simulink model "IEEE9_16b_2"  (R2020a)
settings: Solver=ode15s  StartTime=0.0  StopTime=5  MaxStep=1e-4  RelTol=1e-3
libraries: powerlib x35, sps_avr x3, simulink_extras x2, powerlib_meascontrol x2, simulink x1
settings Model: Creator=Pankaj  LastModifiedBy=ahmed
settings DataIOCC: ReturnWorkspaceOutputs=off
settings DebuggingCC: UnconnectedInputMsg=none  UnconnectedOutputMsg=none  UnconnectedLineMsg=none  ArithmeticOperatorsInVariantConditions=warning
settings SFSimCC: SimUseLocalCustomCode=off  CustomCodeUndefinedFunction=UseInterfaceOnly
settings RTWCC: RTWUseLocalCustomCode=off
settings CodeAppCC: StateflowObjectComments=on
settings SimscapeCC: SimscapeNormalizeSystem=off

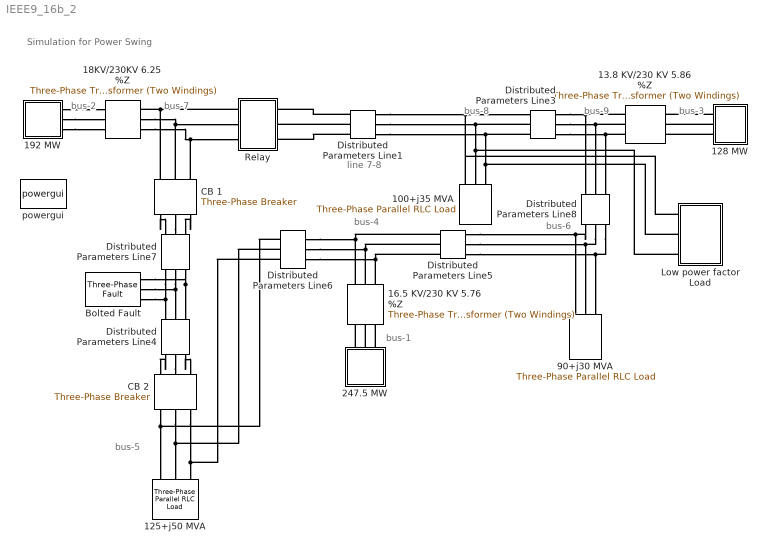
== system IEEE9_16b_2 ==
  note: Simulation for Power Swing
  note: bus-2
  note: bus-7
  note: bus-8
  note: bus-9
  note: bus-1
  note: bus-3
  note: bus-4
  note: bus-6
  note: bus-5
  note: line 7-8
  100+j35 MVA : powerlib/Elements/Three-Phase Parallel RLC Load  LConnTagsString=A|B|C  Configuration=Y (grounded)  NominalVoltage=(230000)*0.993698  Vabc=[1e3 1e3 1e3]  Vabcp=[1e3 1e3 1e3]  NominalFrequency=60  UnbalancedPower=off  ActivePower=100e6  InductivePower=35e6  CapacitivePower=0  Pabc=[10e3 9e3 11e3]  QLabc=[100 90 110]  QCabc=[100 90 110]  Pabcp=[10e3 9e3 11e3]  QLabcp=[100 90 110]  QCabcp=[100 90 110]  Measurements=None  LoadType=constant PQ
  125+j50 MVA : powerlib/Elements/Three-Phase Parallel RLC Load  LConnTagsString=A|B|C  Configuration=Y (grounded)  NominalVoltage=(223027)*1  Vabc=[1e3 1e3 1e3]  Vabcp=[1e3 1e3 1e3]  NominalFrequency=60  UnbalancedPower=off  ActivePower=125e6  InductivePower=50e6  CapacitivePower=0  Pabc=[10e3 9e3 11e3]  QLabc=[100 90 110]  QCabc=[100 90 110]  Pabcp=[10e3 9e3 11e3]  QLabcp=[100 90 110]  QCabcp=[100 90 110]  Measurements=None  LoadType=constant PQ
  128 MW : Subsystem
  13.8 KV/230 KV 5.86 %Z : powerlib/Elements/Three-Phase Transformer (Two Windings)  Winding1Connection=Yg  Winding2Connection=Yg  CoreType=Three single-phase transformers  SetSaturation=off  Hysteresis=off  DataFile='hysteresis'  SetInitialFlux=off  Measurements=None  UNITS=pu  NominalPower=[ 100e6 , 60 ]  Winding1=[13.8e3 , 1e-6 , 0 ]  Winding2=[ 230e3 , 1e-6, 0.0586 ]  Rm=500  Lm=500  L0=0.5  Saturation=[ 0,0 ; 0.0024,1.2 ; 1.0,1.52 ]  InitialFluxes=[ 0.8 , -0.8 , 0.7 ]  BreakLoop=off  DiscreteSolver=Trapezoidal iterative  DataType=off  TransfoNumber=1
  "16.5 KV/230 KV 5.76 %Z     " : powerlib/Elements/Three-Phase Transformer (Two Windings)  Winding1Connection=Yg  Winding2Connection=Yg  CoreType=Three single-phase transformers  SetSaturation=off  Hysteresis=off  DataFile='hysteresis'  SetInitialFlux=off  Measurements=None  UNITS=pu  NominalPower=[ 100e6 , 60 ]  Winding1=[16.5e3 , 1e-6, 0 ]  Winding2=[ 230e3 ,1e-6, 0.0576 ]  Rm=500  Lm=500  L0=0.5  Saturation=[ 0,0 ; 0.0024,1.2 ; 1.0,1.52 ]  InitialFluxes=[ 0.8 , -0.8 , 0.7 ]  BreakLoop=off  DiscreteSolver=Trapezoidal iterative  DataType=off  TransfoNumber=1
  18KV/230KV 6.25 %Z : powerlib/Elements/Three-Phase Transformer (Two Windings)  Winding1Connection=Yg  Winding2Connection=Yg  CoreType=Three single-phase transformers  SetSaturation=off  Hysteresis=off  DataFile='hysteresis'  SetInitialFlux=off  Measurements=None  UNITS=pu  NominalPower=[ 100e6 , 60 ]  Winding1=[ 18e3 , 1e-6 , 0]  Winding2=[ 230e3 , 1e-6, 0.0625 ]  Rm=500  Lm=500  L0=0.5  Saturation=[ 0,0 ; 0.0024,1.2 ; 1.0,1.52 ]  InitialFluxes=[ 0.8 , -0.8 , 0.7 ]  BreakLoop=off  DiscreteSolver=Trapezoidal iterative  DataType=off  TransfoNumber=1
  192 MW : Subsystem
  247.5 MW : Subsystem
  90+j30 MVA : powerlib/Elements/Three-Phase Parallel RLC Load  LConnTagsString=A|B|C  Configuration=Y (grounded)  NominalVoltage=(226177)*0.999999  Vabc=[1e3 1e3 1e3]  Vabcp=[1e3 1e3 1e3]  NominalFrequency=60  UnbalancedPower=off  ActivePower=90e6  InductivePower=30e6  CapacitivePower=0  Pabc=[10e3 9e3 11e3]  QLabc=[100 90 110]  QCabc=[100 90 110]  Pabcp=[10e3 9e3 11e3]  QLabcp=[100 90 110]  QCabcp=[100 90 110]  Measurements=None  LoadType=constant PQ
  Bolted Fault : powerlib/Elements/Three-Phase Fault  InitialStates=0  FaultA=on  FaultB=on  FaultC=on  GroundFault=off  SwitchTimes=0.2  External=off  SwitchStatus=NaN  FaultResistance=1e-6  GroundResistance=0.01  SnubberResistance=1e6  SnubberCapacitance=inf  Measurements=None
  CB 1 : powerlib/Elements/Three-Phase Breaker  InitialState=closed  SwitchA=on  SwitchB=on  SwitchC=on  SwitchTimes=3  External=off  BreakerResistance=0.01  SnubberResistance=1e6  SnubberCapacitance=inf  Measurements=None
  CB 2 : powerlib/Elements/Three-Phase Breaker  InitialState=closed  SwitchA=on  SwitchB=on  SwitchC=on  SwitchTimes=3  External=off  BreakerResistance=0.01  SnubberResistance=1e6  SnubberCapacitance=inf  Measurements=None
  Distributed Parameters Line1 : powerlib/Elements/Distributed Parameters Line  Phases=3  Frequency=60  Resistance=[0.044965 0.11241]  Inductance="[1.01e-3  2.02e-3]"  Capacitance=[12.74e-9 7.751e-9]  Length=100  x1=[-0.0004 -6.82796491334943e-09 72528.4160001859 -218588.479822374;-0.00035 -6.27008684641219e-09 76635.5741816138 -217182.598108978;-0.0003 -5.70998104747418e-09 80715.5041084443 -215699.552452614;-0.00025 -5.14784651945875e-09 84766.7562010016 -214139.869772342;-0.0002 -4.58388298608703e-09 88787.8910687075 -212504.104215993;-0.00015 -4.01829082091706e-09 92777.4800214907 -210792.836963279;-0.0001 -3.45127097615198e-09 96734.1055773932 -209006.676019307;-5e-05 -2.8830249112427e-09 100656.361966195 -207146.255998555]  x2=[-0.0004 -1.1431204063284e-08 62229.765747204 -219715.300074861;-0.00035 -1.09478361575261e-08 66359.9919840522 -218503.333092898;-0.0003 -1.04605785377109e-08 70466.6408317295 -217213.732917117;-0.00025 -9.96960432415053e-09 74548.2532174544 -215846.95773632;-0.0002 -9.47508795764522e-09 78603.3789637815 -214403.493159219;-0.00015 -8.97720513750531e-09 82630.577303842 -212883.852041907;-0.0001 -8.47613275912606e-09 86628.4173932417 -211288.574305635;-5e-05 -7.97204885113761e-09 90595.478818433 -209618.226744989]  x3=[-0.0004 2.47214142457228e-11 142.095952291051 -522.350151915625;-0.00035 2.45249559346704e-11 151.916197843285 -519.579075508434;-0.0003 2.43197840235529e-11 161.682468293792 -516.623395129752;-0.00025 2.41059714089733e-11 171.391293733184 -513.484160918744;-0.0002 2.38835940575356e-11 181.039224662013 -510.162488230377;-0.00015 2.36527309788538e-11 190.622833216359 -506.65955723914;-0.0001 2.34134641974804e-11 200.138714385737 -502.976612519736;-5e-05 2.31658787237637e-11 209.583487222877 -499.114962604885]  x4=[-0.0004 -6.81755980373169e-11 226.230187701687 -1047.93268485817;-0.00035 -6.60199840333111e-11 245.941825546425 -1043.48242296301;-0.0003 -6.38409134433403e-11 265.566081431627 -1038.66141673164;-0.00025 -6.16391604808091e-11 285.095982952621 -1033.47137904461;-0.0002 -5.94155074180612e-11 304.52459122839 -1027.91415389759;-0.00015 -5.71707443084416e-11 323.845003366925 -1021.99171574624;-0.0001 -5.49056687055944e-11 343.05035491779 -1015.70616880461;-5e-05 -5.2621085380096e-11 362.133822311028 -1009.05974629762]  x5=0.000395689524753941  V1=ones(3,3)  V2=ones(3,3)  I1=ones(3,3)  I2=ones(3,3)  nHarmo=1  Measurements=None
  Distributed Parameters Line3 : powerlib/Elements/Distributed Parameters Line  Phases=3  Frequency=60  Resistance=[ 0.062951 0.15737]  Inductance="[ 1.414e-3  3.53e-3]"  Capacitance=[12.74e-9 7.751e-9]  Length=100  x1=[-0.00055 -1.2856259388639e-08 0 0;-0.0005 -1.23855852223811e-08 0 0;-0.00045 -1.19105105166692e-08 58077.4295709002 -220849.203256907;-0.0004 -1.1431204063284e-08 62229.765747204 -219715.300074861;-0.00035 -1.09478361575261e-08 66359.9919840522 -218503.333092898;-0.0003 -1.04605785377109e-08 70466.6408317295 -217213.732917117;-0.00025 -9.96960432415053e-09 74548.2532174544 -215846.95773632;-0.0002 -9.47508795764522e-09 78603.3789637815 -214403.493159219;-0.00015 -8.97720513750531e-09 82630.577303842 -212883.852041907;-0.0001 -8.47613275912606e-09 86628.4173932417 -211288.574305635;-5e-05 -7.97204885113761e-09 90595.478818433 -209618.226744989]  x2=[-0.00055 -1.49760945438105e-08 0 0;-0.0005 -1.45496058699479e-08 0 0;-0.00045 -1.41179477903994e-08 67158.9011993995 -221165.376830188;-0.0004 -1.36812736712252e-08 71315.5829852004 -219860.246936089;-0.00035 -1.32397386606606e-08 75446.9266839443 -218477.001743144;-0.0003 -1.27934996339924e-08 79551.4644488867 -217016.132711783;-0.00025 -1.23427151378221e-08 83627.7379573042 -215478.158881818;-0.0002 -1.18875453337346e-08 87674.2989286288 -213863.626688027;-0.00015 -1.14281519413939e-08 91689.7096390155 -212173.109766011;-0.0001 -1.0964698181085e-08 95672.543432159 -210407.208748382;-5e-05 -1.04973487157221e-08 99621.385226177 -208566.551051363]  x3=[-0.00055 -6.89304608922042e-12 0 0;-0.0005 -6.57772896748363e-12 0 0;-0.00045 -6.26007480996533e-12 133.037448642828 -835.2647228767;-0.0004 -5.94019647767513e-12 148.757241469557 -832.60880210302;-0.00035 -5.61820762186136e-12 164.424181556718 -829.657059386518;-0.0003 -5.2942226436313e-12 180.032702515096 -826.410543467325;-0.00025 -4.96835665330503e-12 195.577258711518 -822.870407817091;-0.0002 -4.64072542951725e-12 211.052327239184 -819.037910229153;-0.00015 -4.31144537808173e-12 226.452409879932 -814.914412371656;-0.0001 -3.98063349063283e-12 241.77203505773 -810.501379303756;-5e-05 -3.64840730305896e-12 257.005759782698 -805.800378955086]  x4=[-0.00055 -4.04271531251667e-11 0 0;-0.0005 -3.95164976157587e-11 0 0;-0.00045 -3.85918020829103e-11 132.207750255798 -502.668253747127;-0.0004 -3.76533950665412e-11 141.658729090772 -500.087037974906;-0.00035 -3.67016099781961e-11 151.059377253824 -497.328143659317;-0.0003 -3.57367849825848e-11 160.406354739424 -494.392551022371;-0.00025 -3.4759262877434e-11 169.69634061098 -491.281303066156;-0.0002 -3.37693909716933e-11 178.926034180746 -487.995505202256;-0.00015 -3.27675209621373e-11 188.092156182545 -484.536324859005;-0.0001 -3.17540088084098e-11 197.191449936875 -480.904991066709;-5e-05 -3.07292146065531e-11 206.220682507993 -477.102794020972]  x5=0.000523077718890797  V1=ones(3,3)  V2=ones(3,3)  I1=ones(3,3)  I2=ones(3,3)  nHarmo=1  Measurements=None
  Distributed Parameters Line4 : powerlib/Elements/Distributed Parameters Line  Phases=3  Frequency=60  Resistance=[ 0.16928 0.4232]  Inductance="[ 2.259e-3  5.64e-3]"  Capacitance=[12.74e-9 7.751e-9]  Length=80  x1=[-0.00055 -1.40561812794253e-08 0 0;-0.0005 -1.36829660387334e-08 0 0;-0.00045 -1.33048893053609e-08 48295.948807218 -217554.641827645;-0.0004 -1.29220854081711e-08 52387.9255838606 -216605.688790323;-0.00035 -1.25346903555658e-08 56461.2891799944 -215579.776783167;-0.0003 -1.21428417871626e-08 60514.5923489297 -214477.270307828;-0.00025 -1.1746678924892e-08 64546.3949713508 -213298.561079608;-0.0002 -1.13463425235325e-08 68555.2645669839 -212044.067888283;-0.00015 -1.09419748207014e-08 72539.7768035502 -210714.23644931;-0.0001 -1.0533719486318e-08 76498.516002825 -209309.539245467;-5e-05 -1.01217215715586e-08 80430.0756436207 -207830.475358982]  x2=[-0.00055 -6.92029081309933e-09 0 0;-0.0005 -6.32833411269307e-09 0 0;-0.00045 -5.73412898530969e-09 64426.420227431 -220200.980450415;-0.0004 -5.13788654920156e-09 68565.4107597344 -218947.522559977;-0.00035 -4.53981864646715e-09 72680.0403280773 -217616.273657318;-0.0003 -3.94013776778453e-09 76768.8470241662 -216207.706728834;-0.00025 -3.33905697691445e-09 80830.3781144513 -214722.322231648;-0.0002 -2.73678983499979e-09 84863.1905562757 -213160.647915798;-0.00015 -2.1335503246883e-09 88865.8515105816 -211523.238636734;-0.0001 -1.52955277410559e-09 92836.938850991 -209810.676158175;-5e-05 -9.25011780705398e-10 96775.0416690807 -208023.568945415]  x3=[-0.00055 -7.55288067688039e-11 0 0;-0.0005 -7.41259584887901e-11 0 0;-0.00045 -7.26967736086847e-11 78.3022662123242 -745.938765685069;-0.0004 -7.12417599110705e-11 92.3481089992822 -744.330373079888;-0.00035 -6.97614343553859e-11 106.361140942839 -742.457523437368;-0.0003 -6.82563228942521e-11 120.33638327947 -740.32088217207;-0.00025 -6.67269602866046e-11 134.268870672118 -737.921208422462;-0.0002 -6.51738899076954e-11 148.153652974353 -735.2593547812;-0.00015 -6.35976635560353e-11 161.985796989138 -732.336266992209;-0.0001 -6.19988412573415e-11 175.760388221566 -729.152983614661;-5e-05 -6.03779910655638e-11 189.472532624964 -725.710635653982]  x4=[-0.00055 4.56513386616241e-11 0 0;-0.0005 4.5308230221681e-11 0 0;-0.00045 4.49490239832806e-11 100.066822114028 -290.202191891929;-0.0004 4.45738475706891e-11 105.51888972623 -288.264531923678;-0.00035 4.41828342822994e-11 110.933466979353 -286.224452939841;-0.0003 4.37761230432709e-11 116.308630099881 -284.082679770765;-0.00025 4.33538583561703e-11 121.642469317951 -281.83997337826;-0.0002 4.29161902496303e-11 126.933089545888 -279.497130585228;-0.00015 4.24632742250451e-11 132.178611051516 -277.054983792557;-0.0001 4.19952712013217e-11 137.377170126022 -274.514400683375;-5e-05 4.15123474577058e-11 142.526919746119 -271.876283914763]  x5=0.000528942431650175  V1=ones(3,3)  V2=ones(3,3)  I1=ones(3,3)  I2=ones(3,3)  nHarmo=1  Measurements=None
  Distributed Parameters Line5 : powerlib/Elements/Distributed Parameters Line  Phases=3  Frequency=60  Resistance=[ 0.08993 0.224825]  Inductance="[ 1.29e-3  3.22e-3]"  Capacitance=[12.74e-9 7.751e-9]  Length=100  x1=[-0.0005 -1.54417229393186e-08 59227.4468730644 -220964.294919318;-0.00045 -1.50769173300264e-08 63381.7481353212 -219808.693934478;-0.0004 -1.47067549637975e-08 67513.5301642651 -218574.995967328;-0.00035 -1.43313673575578e-08 71621.3249574154 -217263.639344882;-0.0003 -1.39508878847366e-08 75703.6730348416 -215875.089985903;-0.00025 -1.35654517278786e-08 79759.1239577106 -214409.841235366;-0.0002 -1.31751958306153e-08 83786.2368436198 -212868.413689177;-0.00015 -1.27802588490086e-08 87783.5808785366 -211251.355009202;-0.0001 -1.23807811022875e-08 91749.7358251591 -209559.23972869;-5e-05 -1.19769045229934e-08 95683.2925275201 -207792.669048144]  x2=[-0.0005 -1.64800198971184e-08 47810.7569296928 -220880.136660959;-0.00045 -1.61471045841858e-08 51965.4999610341 -219939.738829347;-0.0004 -1.58084522818807e-08 56101.7798976792 -218921.197455797;-0.00035 -1.54641833117536e-08 60218.1271390618 -217824.874423211;-0.0003 -1.51144199909305e-08 64313.0791666077 -216651.159249941;-0.00025 -1.47592865886536e-08 68385.18106336 -215400.4689514;-0.0002 -1.43989092821299e-08 72432.9860309045 -214073.247891895;-0.00015 -1.40334161117004e-08 76455.0559034106 -212669.967626748;-0.0001 -1.36629369353481e-08 80449.9616586038 -211191.126734758;-5e-05 -1.32876033825604e-08 84416.2839254919 -209637.25064105]  x3=[-0.0005 -1.39450438340109e-11 90.110530585494 -468.848251260046;-0.00045 -1.36379171260647e-11 98.9315787794445 -467.06652149822;-0.0004 -1.33259449311022e-11 107.717477054529 -465.118845225298;-0.00035 -1.30092380913587e-11 116.465103822925 -463.005914441386;-0.0003 -1.26879091312664e-11 125.171351094496 -460.72847986073;-0.00025 -1.23620722174747e-11 133.833125581041 -458.287350644992;-0.0002 -1.20318431182876e-11 142.447349795329 -455.68339411576;-0.00015 -1.16973391625316e-11 151.010963144515 -452.917535446389;-0.0001 -1.13586791978694e-11 159.520923017552 -449.990757333293;-5e-05 -1.1015983548574e-11 167.974205866218 -446.904099646802]  x4=[-0.0005 -3.93672360983282e-11 134.386791841113 -915.942580841835;-0.00045 -3.87069965166257e-11 151.626950313248 -913.246876554873;-0.0004 -3.80330045233687e-11 168.813236451926 -910.226700001204;-0.00035 -3.73454995847032e-11 185.939544051518 -906.883124235176;-0.0003 -3.66447259678603e-11 202.999788216481 -903.217337213338;-0.00025 -3.59309326543691e-11 219.987907523298 -899.230641372365;-0.0002 -3.52043732515953e-11 236.89786617407 -894.924453166305;-0.00015 -3.44653059026349e-11 253.723656141008 -890.300302563323;-0.0001 -3.3713993194598e-11 270.459299301054 -885.35983250211;-5e-05 -3.29507020653121e-11 287.098849559883 -880.104798308154]  x5=0.000499582025297148  V1=ones(3,3)  V2=ones(3,3)  I1=ones(3,3)  I2=ones(3,3)  nHarmo=1  Measurements=None
  Distributed Parameters Line6 : powerlib/Elements/Distributed Parameters Line  Phases=3  Frequency=60  Resistance=[ 0.0529 0.13225]  Inductance="[ 1.192e-3  2.38e-3]"  Capacitance=[12.74e-9 7.751e-9]  Length=100  x1=[-0.00045 -1.33671750716869e-08 0 0;-0.0004 -1.29840046537664e-08 52388.2213168269 -216603.227745078;-0.00035 -1.25962210808172e-08 56461.5384736403 -215577.310601006;-0.0003 -1.22039621304964e-08 60514.7951146823 -214474.799864975;-0.00025 -1.18073671705413e-08 64546.5511371684 -213296.087253798;-0.0002 -1.14065771092526e-08 68555.3740773815 -212041.591558455;-0.00015 -1.10017343454308e-08 72539.8396196194 -210711.758495291;-0.0001 -1.05929827177822e-08 76498.5321022475 -209307.060547664;-5e-05 -1.01804674538136e-08 80430.0450206764 -207827.996798064]  x2=[-0.00045 -1.50769173300264e-08 0 0;-0.0004 -1.47067549637975e-08 67513.5301642651 -218574.995967328;-0.00035 -1.43313673575578e-08 71621.3249574154 -217263.639344882;-0.0003 -1.39508878847366e-08 75703.6730348416 -215875.089985903;-0.00025 -1.35654517278786e-08 79759.1239577106 -214409.841235366;-0.0002 -1.31751958306153e-08 83786.2368436198 -212868.413689177;-0.00015 -1.27802588490086e-08 87783.5808785366 -211251.355009202;-0.0001 -1.23807811022875e-08 91749.7358251591 -209559.23972869;-5e-05 -1.19769045229934e-08 95683.2925275201 -207792.669048144]  x3=[-0.00045 -2.14191175718911e-11 0 0;-0.0004 -2.11528317147279e-11 113.045801628693 -1046.87113054036;-0.00035 -2.08790303571782e-11 132.757560724253 -1044.55441681095;-0.0003 -2.05978107795606e-11 152.422151690629 -1041.86657787103;-0.00025 -2.03092728978519e-11 172.032587792285 -1038.80856869695;-0.0002 -2.00135192281876e-11 191.581901534652 -1035.38147578482;-0.00015 -1.97106548504382e-11 211.063147139644 -1031.58651676444;-0.0001 -1.94007873708751e-11 230.469403013459 -1027.42503996668;-5e-05 -1.90840268839383e-11 249.79377420579 -1022.89852394442]  x4=[-0.00045 -3.48518737560347e-11 0 0;-0.0004 -3.3860723191614e-11 170.092694709932 -386.073129797578;-0.00035 -3.28575420734751e-11 177.339340108603 -382.798555495363;-0.0003 -3.18426868270926e-11 184.522977684155 -379.387974689121;-0.00025 -3.08165180257032e-11 191.641055124364 -375.842599141972;-0.0002 -2.97794002621957e-11 198.691043410209 -372.163688508968;-0.00015 -2.87317020195732e-11 205.670437714421 -368.352549889537;-0.0001 -2.76737955400325e-11 212.576758291438 -364.410537363085;-5e-05 -2.66060566927085e-11 219.407551358443 -360.339051507892]  x5=0.000429504132692574  V1=ones(3,3)  V2=ones(3,3)  I1=ones(3,3)  I2=ones(3,3)  nHarmo=1  Measurements=None
  Distributed Parameters Line7 : powerlib/Elements/Distributed Parameters Line  Phases=3  Frequency=60  Resistance=[ 0.16928 0.4232]  Inductance="[ 2.259e-3  5.64e-3]"  Capacitance=[12.74e-9 7.751e-9]  Length=20  x1=[-0.00015 -2.13190541884307e-09 88865.8515105816 -211523.238636734;-0.0001 -1.52845584541928e-09 92836.938850991 -209810.676158175;-5e-05 -9.24463218911547e-10 96775.0416690807 -208023.568945415]  x2=[-0.00015 -4.00540707204123e-09 92776.5259316086 -210790.754370917;-0.0001 -3.43782632914382e-09 96733.1124034512 -209004.611780059;-5e-05 -2.86902414292128e-09 100655.330061063 -207144.210845835]  x3=[-0.00015 2.91772913405599e-11 284.591423982608 -715.419057494935;-0.0001 2.89453628397094e-11 298.025372274848 -709.927849901303;-5e-05 2.87031501892687e-11 311.353433571401 -704.184408323007]  x4=[-0.00015 -3.97589260516673e-11 123.975117525793 -290.153181832622;-0.0001 -3.81522539820278e-11 129.422014019475 -287.764895368002;-5e-05 -3.65320265982149e-11 134.822927487834 -285.274367406284]  x5=0.000132235607912544  V1=ones(3,3)  V2=ones(3,3)  I1=ones(3,3)  I2=ones(3,3)  nHarmo=1  Measurements=None
  Distributed Parameters Line8 : powerlib/Elements/Distributed Parameters Line  Phases=3  Frequency=60  Resistance=[ 0.20631 0.5157]  Inductance="[ 2.38e-3  6.09e-3]"  Capacitance=[12.74e-9 7.751e-9]  Length=100  x1=[-0.0007 -1.77519770428368e-08 31036.7644346723 -223854.029074571;-0.00065 -1.74431715104659e-08 35250.5405219156 -223229.267237956;-0.0006 -1.71281685023151e-08 39451.792259961 -222525.193105624;-0.00055 -1.68070799374532e-08 43639.0269640709 -221742.056831762;-0.0005 -1.64800198971184e-08 47810.7569296928 -220880.136660959;-0.00045 -1.61471045841858e-08 51965.4999610341 -219939.738829347;-0.0004 -1.58084522818807e-08 56101.7798976792 -218921.197455797;-0.00035 -1.54641833117536e-08 60218.1271390618 -217824.874423211;-0.0003 -1.51144199909305e-08 64313.0791666077 -216651.159249941;-0.00025 -1.47592865886536e-08 68385.18106336 -215400.4689514;-0.0002 -1.43989092821299e-08 72432.9860309045 -214073.247891895;-0.00015 -1.40334161117004e-08 76455.0559034106 -212669.967626748;-0.0001 -1.36629369353481e-08 80449.9616586038 -211191.126734758;-5e-05 -1.32876033825604e-08 84416.2839254919 -209637.25064105]  x2=[-0.0007 -1.62230383430129e-08 46047.3963086879 -226504.047430459;-0.00065 -1.58129594474007e-08 50308.4541681047 -225595.888989612;-0.0006 -1.53972622825922e-08 54551.6376733053 -224607.577403608;-0.00055 -1.49760945438105e-08 58775.4392413945 -223539.463814848;-0.0005 -1.45496058699479e-08 62978.3581757875 -222391.927719005;-0.00045 -1.41179477903994e-08 67158.9011993995 -221165.376830188;-0.0004 -1.36812736712252e-08 71315.5829852005 -219860.246936089;-0.00035 -1.32397386606606e-08 75446.9266839443 -218477.001743144;-0.0003 -1.27934996339924e-08 79551.4644488867 -217016.132711783;-0.00025 -1.23427151378221e-08 83627.7379573042 -215478.158881818;-0.0002 -1.18875453337346e-08 87674.2989286288 -213863.626688027;-0.00015 -1.14281519413939e-08 91689.7096390155 -212173.109766011;-0.0001 -1.0964698181085e-08 95672.543432159 -210407.208748382;-5e-05 -1.04973487157221e-08 99621.385226177 -208566.551051363]  x3=[-0.0007 -4.18504150647578e-11 24.6100303573918 -669.614087088405;-0.00065 -4.13572954088089e-11 37.2268292493843 -669.031279274382;-0.0006 -4.08494817027289e-11 49.8304016262044 -668.210767832504;-0.00055 -4.03271543703095e-11 62.4162694986001 -667.152844286579;-0.0005 -3.97904989919648e-11 74.9799611676454 -665.857884511807;-0.00045 -3.92397062387955e-11 87.5170128135137 -664.326348601228;-0.0004 -3.8674971804844e-11 100.022970081452 -662.55878070226;-0.00035 -3.80964963375657e-11 112.493389664392 -660.55580882336;-0.0003 -3.75044853665396e-11 124.923840881634 -658.318144610899;-0.00025 -3.68991492304449e-11 137.30990725305 -655.846583096318;-0.0002 -3.62807030023282e-11 149.647188068237 -653.142002413653;-0.00015 -3.56493664131896e-11 161.931299950067 -650.205363487544;-0.0001 -3.50053637739131e-11 174.157878412078 -647.037709691817;-5e-05 -3.43489238955698e-11 186.322579409164 -643.640166478783]  x4=[-0.0007 5.14626612385657e-14 41.4725891803423 -353.789217989042;-0.00065 2.35381322552756e-13 48.1335635245818 -352.944672963745;-0.0006 4.1921635400384e-13 54.7774362428946 -351.974728376731;-0.00055 6.02902439880495e-13 61.4018467989396 -350.879728844695;-0.0005 7.86374317391051e-13 68.0044415711891 -349.660063415755;-0.00045 9.69566799851051e-13 74.5828746891595 -348.316165431231;-0.0004 1.15241479984377e-12 81.134808866888 -346.848512371678;-0.00035 1.33485335234547e-12 87.6579162333591 -345.257625687239;-0.0003 1.51681763780714e-12 94.149879159586 -343.544070612379;-0.00025 1.6982430051846e-12 100.608391082053 -341.708455965056;-0.0002 1.8790649949087e-12 107.031157322228 -339.751433930413;-0.00015 2.05921936178751e-12 113.415895901847 -337.673699829062;-0.0001 2.23864209783228e-12 119.760338353696 -335.475991870034;-5e-05 2.41726945499926e-12 126.06223052758 -333.159090888504]  x5=0.000687048688231045  V1=ones(3,3)  V2=ones(3,3)  I1=ones(3,3)  I2=ones(3,3)  nHarmo=1  Measurements=None
  Low power factor Load : Subsystem
  Relay : Subsystem
  powergui : powerlib/powergui  Priority=1  SimulationMode=Discrete  SampleTime=50e-6  frequency=60  Iterations=50  frequencyindice=60  Pbase=100e6  ErrMax=0.0001  UnitsV=kV  UnitsW=MW  buscounter=0  FunctionMessages=off  echomessages=off  EnableUseOfTLC=off  CurrentSourceSwitches=off  DisableSnubberDevices=off  DisableRonSwitches=off  DisableVfSwitches=off  DisplayEquations=off  AutomaticDiscreteSolvers=off  SolverType=Tustin/Backward Euler (TBE)  Interpol=off  ExternalGateDelay=off  methode=off  Ts=100  x0status=blocks  SPID=on  SwTol=0  HookPort=off  NonlinearTolerance=1e-4  nMaxIteration=100  ContinueOnMaxIteration=off  RestoreLinks=warning  ResistiveCurrentMeasurement=off  Frange=[0:2:500]  Ylog=off  Xlog=on  ShowGrid=off  save=off  variable=ZData  structure=0  ZoomFFT=off  StartTime=0.0  cycles=1  DisplayStyle=1  fundamental=60  FreqAxis=off  MaxFrequency=1000  frequencyindicesteady=1  RmsSteady=1  display=off
  connections:
  Distributed Parameters Line1/RConn1 -- 100+j35 MVA/LConn1 -- Low power factor Load/RConn1 -- Distributed Parameters Line3/LConn1
  Distributed Parameters Line1/RConn2 -- Low power factor Load/RConn3 -- 100+j35 MVA/LConn2 -- Distributed Parameters Line3/LConn2
  Distributed Parameters Line1/RConn3 -- Distributed Parameters Line3/LConn3 -- 100+j35 MVA/LConn3 -- Low power factor Load/RConn2
  Distributed Parameters Line5/RConn1 -- Distributed Parameters Line8/LConn1 -- 90+j30 MVA/LConn1
  Distributed Parameters Line5/RConn3 -- Distributed Parameters Line8/LConn3 -- 90+j30 MVA/LConn3
  Distributed Parameters Line3/RConn1 -- 13.8 KV/230 KV 5.86 %Z/RConn1 -- Distributed Parameters Line8/RConn1
  Distributed Parameters Line3/RConn2 -- 13.8 KV/230 KV 5.86 %Z/RConn2 -- Distributed Parameters Line8/RConn2
  Distributed Parameters Line3/RConn3 -- 13.8 KV/230 KV 5.86 %Z/RConn3 -- Distributed Parameters Line8/RConn3
  Relay/LConn1 -- CB 1/RConn1 -- 18KV/230KV 6.25 %Z/RConn1
  18KV/230KV 6.25 %Z/RConn2 -- CB 1/RConn2 -- Relay/LConn2
  18KV/230KV 6.25 %Z/RConn3 -- Relay/LConn3 -- CB 1/RConn3
  Distributed Parameters Line5/RConn2 -- Distributed Parameters Line8/LConn2 -- 90+j30 MVA/LConn2
  Distributed Parameters Line6/RConn1 -- Distributed Parameters Line5/LConn1 -- "16.5 KV/230 KV 5.76 %Z     "/RConn1
  Distributed Parameters Line6/RConn2 -- Distributed Parameters Line5/LConn2 -- "16.5 KV/230 KV 5.76 %Z     "/RConn2
  Distributed Parameters Line6/RConn3 -- Distributed Parameters Line5/LConn3 -- "16.5 KV/230 KV 5.76 %Z     "/RConn3
  247.5 MW/RConn1 -- "16.5 KV/230 KV 5.76 %Z     "/LConn1
  247.5 MW/RConn2 -- "16.5 KV/230 KV 5.76 %Z     "/LConn2
  247.5 MW/RConn3 -- "16.5 KV/230 KV 5.76 %Z     "/LConn3
  128 MW/RConn1 -- 13.8 KV/230 KV 5.86 %Z/LConn1
  128 MW/RConn2 -- 13.8 KV/230 KV 5.86 %Z/LConn2
  128 MW/RConn3 -- 13.8 KV/230 KV 5.86 %Z/LConn3
  192 MW/RConn1 -- 18KV/230KV 6.25 %Z/LConn1
  192 MW/RConn2 -- 18KV/230KV 6.25 %Z/LConn2
  192 MW/RConn3 -- 18KV/230KV 6.25 %Z/LConn3
  Distributed Parameters Line1/LConn1 -- Relay/RConn1
  Distributed Parameters Line1/LConn2 -- Relay/RConn2
  Distributed Parameters Line1/LConn3 -- Relay/RConn3
  Distributed Parameters Line7/LConn1 -- Distributed Parameters Line4/RConn1 -- Bolted Fault/LConn1
  Distributed Parameters Line7/LConn2 -- Distributed Parameters Line4/RConn2 -- Bolted Fault/LConn2
  Distributed Parameters Line7/LConn3 -- Distributed Parameters Line4/RConn3 -- Bolted Fault/LConn3
  CB 1/LConn2 -- Distributed Parameters Line7/RConn2
  CB 1/LConn1 -- Distributed Parameters Line7/RConn1
  CB 1/LConn3 -- Distributed Parameters Line7/RConn3
  Distributed Parameters Line4/LConn2 -- CB 2/RConn2
  Distributed Parameters Line4/LConn1 -- CB 2/RConn1
  Distributed Parameters Line4/LConn3 -- CB 2/RConn3
  CB 2/LConn2 -- Distributed Parameters Line6/LConn2 -- 125+j50 MVA/LConn2
  CB 2/LConn1 -- Distributed Parameters Line6/LConn1 -- 125+j50 MVA/LConn1
  CB 2/LConn3 -- Distributed Parameters Line6/LConn3 -- 125+j50 MVA/LConn3

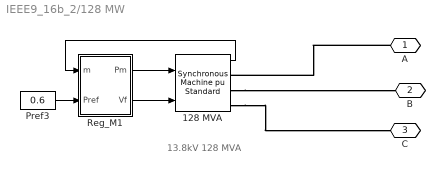
== system IEEE9_16b_2/128 MW ==
  note: 13.8kV 128 MVA
  128 MVA : powerlib/Machines/Synchronous Machine pu Standard  PresetModel=No  MechanicalLoad=Mechanical power Pm  ShowDetailedParameters=on  RotorType=Salient-pole  Units=per unit standard parameters  MeasurementBus=off  NominalParameters="[128e6  13800   60 ]"  Reactances1=[ 31 32 33 34 35 36 37 ]  Reactances2=[ 1.305, 0.296, 0.252, 0.474, 0.243, 0.18 ]  dAxisTimeConstants=Short-circuit  qAxisTimeConstants=Open-circuit  TimeConstants1=[]  TimeConstants2=[]  TimeConstants3=[]  TimeConstants4=[]  TimeConstants5=[ 1.01, 0.053, 0.1 ]  TimeConstants6=[]  TimeConstants7=[]  TimeConstants8=[]  StatorResistance=2.8544e-3  Mechanical="[20 0  32]"  PolePairs=32  InitialConditions=[0 -74.5248 0.603223 0.603223 0.603223 5.08525 -114.915 125.085 1.10339]  SetSaturation=off  Saturation=[0.6404,0.7127,0.8441,0.9214,0.9956,1.082,1.19,1.316,1.457;0.7,0.7698,0.8872,0.9466,0.9969,1.046,1.1,1.151,1.201]  LoadFlowParameters=[1 500000000 0 0 0]  TsPowergui=0  TsBlock=-1  IterativeModel=Trapezoidal non iterative  IterativeDiscreteModel=Trapezoidal non iterative  BusType=PV  Pref=0.6*128e6  Qref=0  Qmin=-Inf  Qmax=Inf  PLF=0  QLF=0
      settings: AttributesFormatString=\n\n
  Pref3 : Constant  Value=0.6
  Reg_M1 : Subsystem
  A : PMIOPort  Side=Right
  B : PMIOPort  Port=2  Side=Right
  C : PMIOPort  Port=3  Side=Right
  wires:
  Reg_M1/1(Pm) -> 128 MVA/1
  Reg_M1/2(Vf) -> 128 MVA/2
  Pref3/1 -> Reg_M1/2(Pref)
  128 MVA/1 -> Reg_M1/1(m)
  connections:
  A/RConn1 -- 128 MVA/RConn1
  128 MVA/RConn2 -- B/RConn1
  128 MVA/RConn3 -- C/RConn1

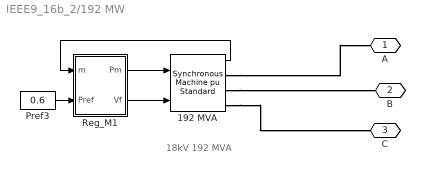
== system IEEE9_16b_2/192 MW ==
  note: 18kV 192 MVA
  192 MVA : powerlib/Machines/Synchronous Machine pu Standard  PresetModel=No  MechanicalLoad=Mechanical power Pm  ShowDetailedParameters=on  RotorType=Salient-pole  Units=per unit standard parameters  MeasurementBus=off  NominalParameters="[192e6  18000   60 ]"  Reactances1=[ 31 32 33 34 35 36 37 ]  Reactances2=[ 1.305, 0.296, 0.252, 0.474, 0.243, 0.18 ]  dAxisTimeConstants=Short-circuit  qAxisTimeConstants=Open-circuit  TimeConstants1=[]  TimeConstants2=[]  TimeConstants3=[]  TimeConstants4=[]  TimeConstants5=[ 1.01, 0.053, 0.1 ]  TimeConstants6=[]  TimeConstants7=[]  TimeConstants8=[]  StatorResistance=2.8544e-3  Mechanical="[20 0  32]"  PolePairs=32  InitialConditions=[0 -73.0594 0.600015 0.600015 0.600015 0.71576 -119.284 120.716 1.18255]  SetSaturation=off  Saturation=[0.6404,0.7127,0.8441,0.9214,0.9956,1.082,1.19,1.316,1.457;0.7,0.7698,0.8872,0.9466,0.9969,1.046,1.1,1.151,1.201]  LoadFlowParameters=[1 500000000 0 0 0]  TsPowergui=0  TsBlock=-1  IterativeModel=Trapezoidal non iterative  IterativeDiscreteModel=Trapezoidal non iterative  BusType=PV  Pref=0.6*192e6  Qref=0  Qmin=-Inf  Qmax=Inf  PLF=0  QLF=0
      settings: AttributesFormatString=\n\n
  Pref3 : Constant  Value=0.6
  Reg_M1 : Subsystem
  A : PMIOPort  Side=Right
  B : PMIOPort  Port=2  Side=Right
  C : PMIOPort  Port=3  Side=Right
  wires:
  Reg_M1/1(Pm) -> 192 MVA/1
  192 MVA/1 -> Reg_M1/1(m)
  Reg_M1/2(Vf) -> 192 MVA/2
  Pref3/1 -> Reg_M1/2(Pref)
  connections:
  192 MVA/RConn1 -- A/RConn1
  192 MVA/RConn3 -- C/RConn1
  192 MVA/RConn2 -- B/RConn1

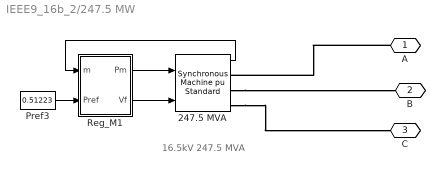
== system IEEE9_16b_2/247.5 MW ==
  note: 16.5kV 247.5 MVA
  247.5 MVA : powerlib/Machines/Synchronous Machine pu Standard  PresetModel=No  MechanicalLoad=Mechanical power Pm  ShowDetailedParameters=on  RotorType=Salient-pole  Units=per unit standard parameters  MeasurementBus=off  NominalParameters="[247.5e6  16500   60 ]"  Reactances1=[ 31 32 33 34 35 36 37 ]  Reactances2=[ 1.305, 0.296, 0.252, 0.474, 0.243, 0.18 ]  dAxisTimeConstants=Short-circuit  qAxisTimeConstants=Open-circuit  TimeConstants1=[]  TimeConstants2=[]  TimeConstants3=[]  TimeConstants4=[]  TimeConstants5=[ 1.01, 0.053, 0.1 ]  TimeConstants6=[]  TimeConstants7=[]  TimeConstants8=[]  StatorResistance=2.8544e-3  Mechanical=[20 0 32]  PolePairs=32  InitialConditions=[0 -76.6925 0.514814 0.514814 0.514814 -5.74321 -125.743 114.257 1.19383]  SetSaturation=off  Saturation=[0.6404,0.7127,0.8441,0.9214,0.9956,1.082,1.19,1.316,1.457;0.7,0.7698,0.8872,0.9466,0.9969,1.046,1.1,1.151,1.201]  LoadFlowParameters=[1 500000000 0 0 0]  TsPowergui=0  TsBlock=-1  IterativeModel=Trapezoidal non iterative  IterativeDiscreteModel=Trapezoidal non iterative  BusType=swing  Pref=5e+008  Qref=0  Qmin=-Inf  Qmax=Inf  PLF=0  QLF=0
      settings: AttributesFormatString=\n\n
  Pref3 : Constant  Value=0.51223
  Reg_M1 : Subsystem
  A : PMIOPort  Side=Right
  B : PMIOPort  Port=2  Side=Right
  C : PMIOPort  Port=3  Side=Right
  wires:
  Reg_M1/1(Pm) -> 247.5 MVA/1
  Reg_M1/2(Vf) -> 247.5 MVA/2
  Pref3/1 -> Reg_M1/2(Pref)
  247.5 MVA/1 -> Reg_M1/1(m)
  connections:
  A/RConn1 -- 247.5 MVA/RConn1
  247.5 MVA/RConn2 -- B/RConn1
  247.5 MVA/RConn3 -- C/RConn1

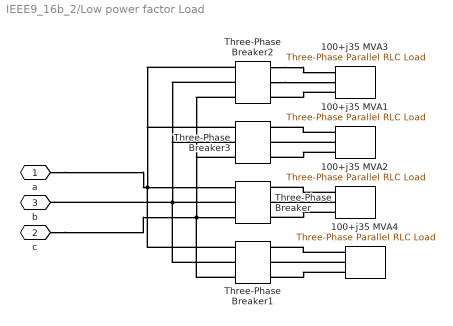
== system IEEE9_16b_2/Low power factor Load ==
  100+j35 MVA{1..4} (4 alike) : powerlib/Elements/Three-Phase Parallel RLC Load  LConnTagsString=A|B|C  Configuration=Y (grounded)  NominalVoltage=(230000)*0.993698  Vabc=[1e3 1e3 1e3]  Vabcp=[1e3 1e3 1e3]  NominalFrequency=60  UnbalancedPower=off  ActivePower=50e6  InductivePower=60e6  CapacitivePower=0  Pabc=[10e3 9e3 11e3]  QLabc=[100 90 110]  QCabc=[100 90 110]  Pabcp=[10e3 9e3 11e3]  QLabcp=[100 90 110]  QCabcp=[100 90 110]  Measurements=None  LoadType=constant PQ
  Three-Phase Breaker : powerlib/Elements/Three-Phase Breaker  InitialState=open  SwitchA=on  SwitchB=on  SwitchC=on  SwitchTimes=0.5  External=off  BreakerResistance=0.01  SnubberResistance=1e6  SnubberCapacitance=inf  Measurements=None
  Three-Phase Breaker1 : powerlib/Elements/Three-Phase Breaker  InitialState=open  SwitchA=on  SwitchB=on  SwitchC=on  SwitchTimes=0.6  External=off  BreakerResistance=0.01  SnubberResistance=1e6  SnubberCapacitance=inf  Measurements=None
  Three-Phase Breaker2 : powerlib/Elements/Three-Phase Breaker  InitialState=open  SwitchA=on  SwitchB=on  SwitchC=on  SwitchTimes=0.1  External=off  BreakerResistance=0.01  SnubberResistance=1e6  SnubberCapacitance=inf  Measurements=None
  Three-Phase Breaker3 : powerlib/Elements/Three-Phase Breaker  InitialState=open  SwitchA=on  SwitchB=on  SwitchC=on  SwitchTimes=0.15  External=off  BreakerResistance=0.01  SnubberResistance=1e6  SnubberCapacitance=inf  Measurements=None
  a : PMIOPort  Side=Right
  c : PMIOPort  Port=2  Side=Right
  b : PMIOPort  Port=3  Side=Right
  connections:
  100+j35 MVA2/LConn3 -- Three-Phase Breaker/LConn3
  100+j35 MVA2/LConn2 -- Three-Phase Breaker/LConn2
  100+j35 MVA2/LConn1 -- Three-Phase Breaker/LConn1
  a/RConn1 -- Three-Phase Breaker1/RConn1 -- Three-Phase Breaker3/RConn1 -- Three-Phase Breaker2/RConn1 -- Three-Phase Breaker/RConn1
  Three-Phase Breaker/RConn2 -- Three-Phase Breaker3/RConn2 -- Three-Phase Breaker2/RConn2 -- Three-Phase Breaker1/RConn2 -- b/RConn1
  c/RConn1 -- Three-Phase Breaker1/RConn3 -- Three-Phase Breaker3/RConn3 -- Three-Phase Breaker2/RConn3 -- Three-Phase Breaker/RConn3
  100+j35 MVA4/LConn1 -- Three-Phase Breaker1/LConn1
  100+j35 MVA4/LConn3 -- Three-Phase Breaker1/LConn3
  100+j35 MVA4/LConn2 -- Three-Phase Breaker1/LConn2
  100+j35 MVA1/LConn2 -- Three-Phase Breaker3/LConn2
  100+j35 MVA1/LConn3 -- Three-Phase Breaker3/LConn3
  100+j35 MVA1/LConn1 -- Three-Phase Breaker3/LConn1
  Three-Phase Breaker2/LConn1 -- 100+j35 MVA3/LConn1
  100+j35 MVA3/LConn3 -- Three-Phase Breaker2/LConn3
  Three-Phase Breaker2/LConn2 -- 100+j35 MVA3/LConn2

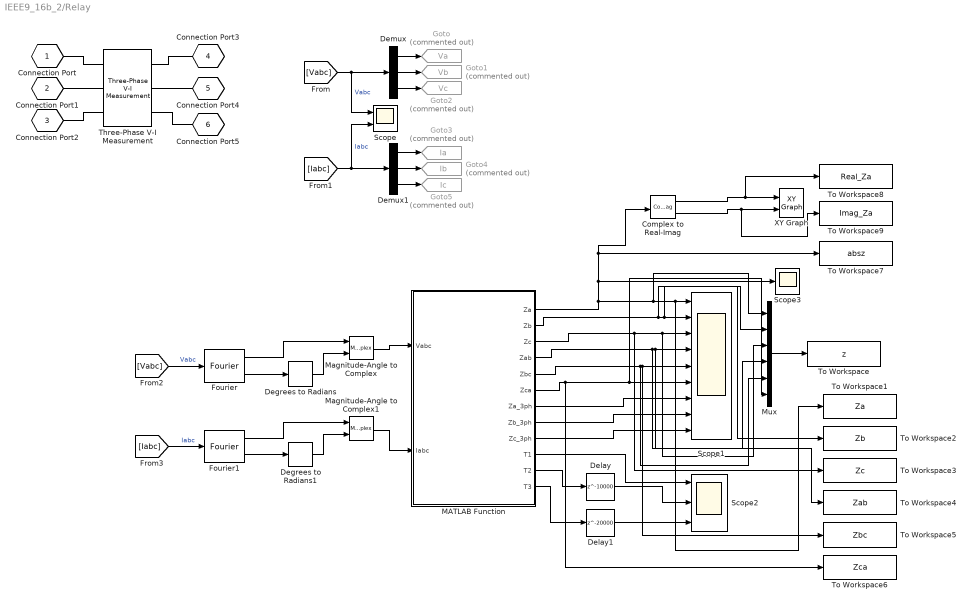
== system IEEE9_16b_2/Relay ==
  Complex to Real-Imag : ComplexToRealImag
  Degrees to Radians : simulink_extras/Transformations/Degrees to Radians
  Degrees to Radians1 : simulink_extras/Transformations/Degrees to Radians
  Delay : Delay  DelayLength=10000  SampleTime=50e-6
  Delay1 : Delay  DelayLength=20000  SampleTime=50e-6
  Demux : Demux  Outputs=3
  Demux1 : Demux  Outputs=3
  Fourier : powerlib_meascontrol/Measurements/Fourier  Freq=60  n=1  InInit=[0, 0]  Ts=0
  Fourier1 : powerlib_meascontrol/Measurements/Fourier  Freq=60  n=1  InInit=[0, 0]  Ts=0
  Goto : Goto  Commented=on  GotoTag=Va  TagVisibility=global
  Goto1 : Goto  Commented=on  GotoTag=Vb  TagVisibility=global
  Goto2 : Goto  Commented=on  GotoTag=Vc  TagVisibility=global
  Goto3 : Goto  Commented=on  GotoTag=Ia  TagVisibility=global
  Goto4 : Goto  Commented=on  GotoTag=Ib  TagVisibility=global
  Goto5 : Goto  Commented=on  GotoTag=Ic  TagVisibility=global
  MATLAB Function : MATLAB Function  TreatAsAtomicUnit=on
  Magnitude-Angle to Complex : MagnitudeAngleToComplex
  Magnitude-Angle to Complex1 : MagnitudeAngleToComplex
  Mux : Mux  Inputs=6
  Scope : Scope  NumInputPorts=2
  Scope1 : Scope  NumInputPorts=9
  Scope2 : Scope  NumInputPorts=3
  Scope3 : Scope
  Three-Phase V-I Measurement : powerlib/Measurements/Three-Phase V-I Measurement  VoltageMeasurement=phase-to-ground  SetLabelV=on  LabelV=Vabc  Vpu=off  VpuLL=off  CurrentMeasurement=yes  SetLabelI=on  LabelI=Iabc  Ipu=off  Pbase=100e6  Vbase=500e3  OutputType=Complex  PhasorSimulation=off  PSBequivalent=0
  To Workspace : ToWorkspace  VariableName=z  SampleTime=-1
  To Workspace1 : ToWorkspace  VariableName=Za  SampleTime=-1
  To Workspace2 : ToWorkspace  VariableName=Zb  SampleTime=-1
  To Workspace3 : ToWorkspace  VariableName=Zc  SampleTime=-1
  To Workspace4 : ToWorkspace  VariableName=Zab  SampleTime=-1
  To Workspace5 : ToWorkspace  VariableName=Zbc  SampleTime=-1
  To Workspace6 : ToWorkspace  VariableName=Zca  SampleTime=-1
  To Workspace7 : ToWorkspace  VariableName=absz  SampleTime=-1
  To Workspace8 : ToWorkspace  VariableName=Real_Za  SampleTime=-1
      settings: Save2DSignal=2-D array (concatenate along first dimension)
  To Workspace9 : ToWorkspace  VariableName=Imag_Za  SampleTime=-1
      settings: Save2DSignal=2-D array (concatenate along first dimension)
  XY Graph : simulink/Sinks/XY Graph  xmin=-500  xmax=1000  ymin=-200  ymax=500  st=1e-3
  Connection Port : PMIOPort  Tag=PMCPort  Side=Left
  Connection Port1 : PMIOPort  Tag=PMCPort  Port=2  Side=Left
  Connection Port2 : PMIOPort  Tag=PMCPort  Port=3  Side=Left
  Connection Port3 : PMIOPort  Tag=PMCPort  Port=4  Side=Right
  Connection Port4 : PMIOPort  Tag=PMCPort  Port=5  Side=Right
  Connection Port5 : PMIOPort  Tag=PMCPort  Port=6  Side=Right
  wires:
  Demux1/3 -> Goto5/1
  Demux1/1 -> Goto3/1
  Demux/3 -> Goto2/1
  Demux/1 -> Goto/1
  Demux/2 -> Goto1/1
  [Iabc] -> Scope/2, Demux1/1  "Iabc"
  [Vabc] -> Scope/1, Demux/1  "Vabc"
  Demux1/2 -> Goto4/1
  MATLAB Function/1(Za) -> To Workspace7/1, Complex to Real-Imag/1, Scope3/1, Mux/1, To Workspace1/1, Scope1/1
  MATLAB Function/2(Zb) -> To Workspace2/1, Mux/2, Scope1/2
  MATLAB Function/3(Zc) -> To Workspace3/1, Mux/3, Scope1/3
  MATLAB Function/4(Zab) -> To Workspace4/1, Scope1/4, Mux/4
  MATLAB Function/5(Zbc) -> To Workspace5/1, Scope1/5, Mux/5
  MATLAB Function/6(Zca) -> To Workspace6/1, Mux/6, Scope1/6
  MATLAB Function/10(T1) -> Scope2/1
  Fourier/2 -> Degrees to Radians/1
  Degrees to Radians/1 -> Magnitude-Angle to Complex/2
  Fourier/1 -> Magnitude-Angle to Complex/1
  Magnitude-Angle to Complex/1 -> MATLAB Function/1(Vabc)
  [Vabc] -> Fourier/1  "Vabc"
  Fourier1/1 -> Magnitude-Angle to Complex1/1
  Degrees to Radians1/1 -> Magnitude-Angle to Complex1/2
  Fourier1/2 -> Degrees to Radians1/1
  [Iabc] -> Fourier1/1  "Iabc"
  Magnitude-Angle to Complex1/1 -> MATLAB Function/2(Iabc)
  MATLAB Function/11(T2) -> Delay/1
  MATLAB Function/12(T3) -> Delay1/1
  Delay/1 -> Scope2/2
  Delay1/1 -> Scope2/3
  MATLAB Function/7(Za_3ph) -> Scope1/7
  MATLAB Function/8(Zb_3ph) -> Scope1/8
  MATLAB Function/9(Zc_3ph) -> Scope1/9
  Complex to Real-Imag/1 -> To Workspace8/1, XY Graph/1
  Complex to Real-Imag/2 -> To Workspace9/1, XY Graph/2
  Mux/1 -> To Workspace/1
  connections:
  Connection Port/RConn1 -- Three-Phase V-I Measurement/LConn1
  Connection Port1/RConn1 -- Three-Phase V-I Measurement/LConn2
  Connection Port2/RConn1 -- Three-Phase V-I Measurement/LConn3
  Connection Port3/RConn1 -- Three-Phase V-I Measurement/RConn1
  Connection Port4/RConn1 -- Three-Phase V-I Measurement/RConn2
  Connection Port5/RConn1 -- Three-Phase V-I Measurement/RConn3

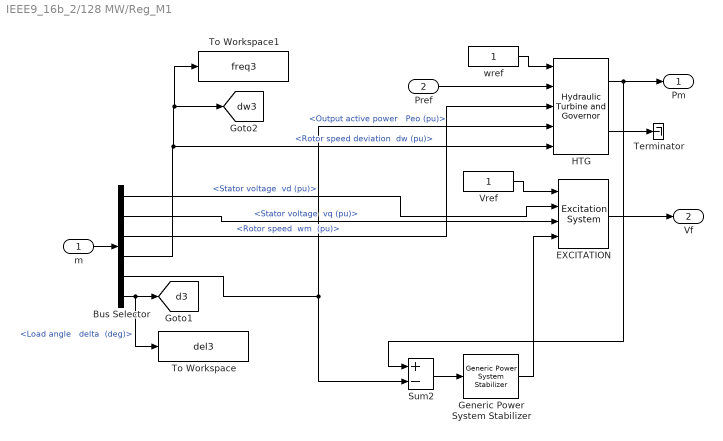
== system IEEE9_16b_2/128 MW/Reg_M1 ==
  m : Inport
  Pref : Inport  Port=2
  Bus Selector : BusSelector  OutputSignals="dq0 components.Stator voltage  vd (pu),dq0 components.Stator voltage  vq (pu),Mechanical.Rotor speed  wm  (pu),Mechanical.Rotor speed deviation  dw (pu),Output active power   Peo (pu),Load angle   delta  (deg)"
  EXCITATION : sps_avr/Excitation System  tr=20e-3  reg=[ 200, 0.001 ]  exc=[ 1, 0 ]  tgr=[ 0, 0 ]  damp=[ 0.001, 0.1 ]  sat=[ 0, 0 ]  lim="[ 0,  7, 0 ]"  v0=[1 1.1034]
      settings: SourceProductBaseCode=PS
  Generic Power System Stabilizer : powerlib/Machines/Generic Power System Stabilizer  Tsensor=15e-3  K=2.5  Twashout=1  Tleadlag1="[0.06  1]"  Tleadlag2="[0  0]"  VSlimits=[-0.15 0.15]  Vinit=0  Plot_On=off  MagdB_On=on  FreqRange=logspace(-2,2,500)
      settings: SourceProductBaseCode=PS
  HTG : powerlib/Machines/Hydraulic Turbine and Governor  sm="[ 10/3  0.07 ]"  gate="[  0.01  0.97518  -0.1  0.1 ]"  reg="[  0.05  1.163  0.105  0  0.01  ]"  hyd="[  0  2.67  ]"  dref=0  po=0.60104
      settings: SourceProductBaseCode=PS
  Sum2 : Sum  Inputs=+-  InputSameDT=on  SaturateOnIntegerOverflow=on  OutDataTypeStr=Inherit: Same as first input
  Terminator : Terminator
  To Workspace : ToWorkspace  VariableName=del3  SampleTime=-1
  To Workspace1 : ToWorkspace  VariableName=freq3  SampleTime=-1
  Vref : Constant
  wref : Constant
  Pm : Outport  InitialOutput=0
  Vf : Outport  Port=2  InitialOutput=0
  tag scope: d3=global, dw3=global
  wires:
  HTG/2 -> Terminator/1
  Vref/1 -> EXCITATION/1
  m/1 -> Bus Selector/1
  Bus Selector/4 -> To Workspace1/1, [dw3], HTG/5  "<Rotor speed deviation  dw (pu)>"
  Bus Selector/5 -> HTG/4, Sum2/2  "<Output active power   Peo (pu)>"
  Bus Selector/3 -> HTG/3  "<Rotor speed  wm  (pu)>"
  Pref/1 -> HTG/2
  wref/1 -> HTG/1
  HTG/1 -> Pm/1, Sum2/1
  Bus Selector/2 -> EXCITATION/3  "<Stator voltage  vq (pu)>"
  EXCITATION/1 -> Vf/1
  Bus Selector/1 -> EXCITATION/2  "<Stator voltage  vd (pu)>"
  Generic Power System Stabilizer/1 -> EXCITATION/4
  Sum2/1 -> Generic Power System Stabilizer/1
  Bus Selector/6 -> To Workspace/1, [d3]  "<Load angle   delta  (deg)>"

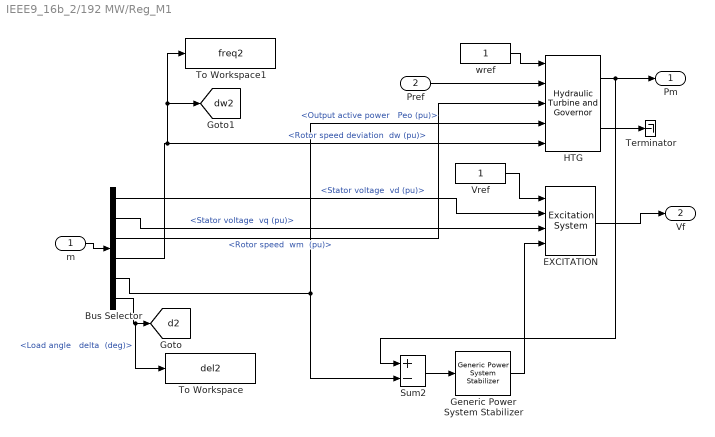
== system IEEE9_16b_2/192 MW/Reg_M1 ==
  m : Inport
  Pref : Inport  Port=2
  Bus Selector : BusSelector  OutputSignals="dq0 components.Stator voltage  vd (pu),dq0 components.Stator voltage  vq (pu),Mechanical.Rotor speed  wm  (pu),Mechanical.Rotor speed deviation  dw (pu),Output active power   Peo (pu),Load angle   delta  (deg)"
  EXCITATION : sps_avr/Excitation System  tr=20e-3  reg=[ 200, 0.001 ]  exc=[ 1, 0 ]  tgr=[ 0, 0 ]  damp=[ 0.001, 0.1 ]  sat=[ 0, 0 ]  lim="[ 0,  7, 0 ]"  v0=[1 1.1826]
      settings: SourceProductBaseCode=PS
  Generic Power System Stabilizer : powerlib/Machines/Generic Power System Stabilizer  Tsensor=15e-3  K=2.5  Twashout=1  Tleadlag1="[0.06  1]"  Tleadlag2="[0  0]"  VSlimits=[-0.15 0.15]  Vinit=0  Plot_On=off  MagdB_On=on  FreqRange=logspace(-2,2,500)
      settings: SourceProductBaseCode=PS
  HTG : powerlib/Machines/Hydraulic Turbine and Governor  sm="[ 10/3  0.07 ]"  gate="[  0.01  0.97518  -0.1  0.1 ]"  reg="[  0.05  1.163  0.105  0  0.01  ]"  hyd="[  0  2.67  ]"  dref=0  po=0.60103
      settings: SourceProductBaseCode=PS
  Sum2 : Sum  Inputs=+-  InputSameDT=on  SaturateOnIntegerOverflow=on  OutDataTypeStr=Inherit: Same as first input
  Terminator : Terminator
  To Workspace : ToWorkspace  VariableName=del2  SampleTime=-1
  To Workspace1 : ToWorkspace  VariableName=freq2  SampleTime=-1
  Vref : Constant
  wref : Constant
  Pm : Outport  InitialOutput=0
  Vf : Outport  Port=2  InitialOutput=0
  tag scope: d2=global, dw2=global
  wires:
  HTG/2 -> Terminator/1
  Vref/1 -> EXCITATION/1
  m/1 -> Bus Selector/1
  Bus Selector/4 -> To Workspace1/1, [dw2], HTG/5  "<Rotor speed deviation  dw (pu)>"
  Bus Selector/5 -> HTG/4, Sum2/2  "<Output active power   Peo (pu)>"
  Bus Selector/3 -> HTG/3  "<Rotor speed  wm  (pu)>"
  Pref/1 -> HTG/2
  wref/1 -> HTG/1
  HTG/1 -> Pm/1, Sum2/1
  Bus Selector/2 -> EXCITATION/3  "<Stator voltage  vq (pu)>"
  EXCITATION/1 -> Vf/1
  Bus Selector/1 -> EXCITATION/2  "<Stator voltage  vd (pu)>"
  Generic Power System Stabilizer/1 -> EXCITATION/4
  Sum2/1 -> Generic Power System Stabilizer/1
  Bus Selector/6 -> To Workspace/1, [d2]  "<Load angle   delta  (deg)>"

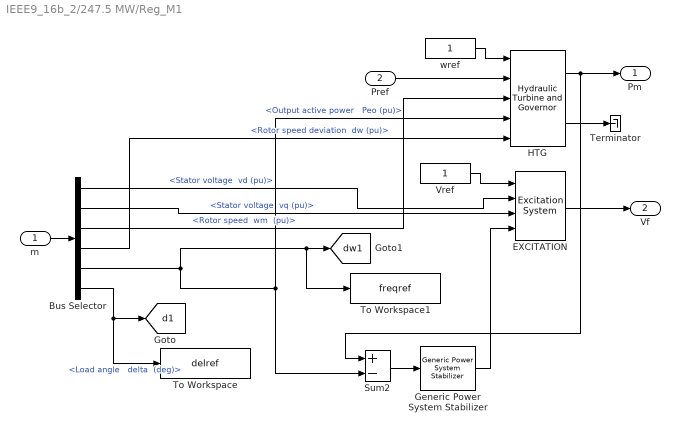
== system IEEE9_16b_2/247.5 MW/Reg_M1 ==
  m : Inport
  Pref : Inport  Port=2
  Bus Selector : BusSelector  OutputSignals="dq0 components.Stator voltage  vd (pu),dq0 components.Stator voltage  vq (pu),Mechanical.Rotor speed  wm  (pu),Mechanical.Rotor speed deviation  dw (pu),Output active power   Peo (pu),Load angle   delta  (deg)"
  EXCITATION : sps_avr/Excitation System  tr=20e-3  reg=[ 200, 0.001 ]  exc=[ 1, 0 ]  tgr=[ 0, 0 ]  damp=[ 0.001, 0.1 ]  sat=[ 0, 0 ]  lim="[ 0,  7, 0 ]"  v0=[1 1.1938]
      settings: SourceProductBaseCode=PS
  Generic Power System Stabilizer : powerlib/Machines/Generic Power System Stabilizer  Tsensor=15e-3  K=2.5  Twashout=1  Tleadlag1="[0.06  1]"  Tleadlag2="[0  0]"  VSlimits=[-0.15 0.15]  Vinit=0  Plot_On=off  MagdB_On=on  FreqRange=logspace(-2,2,500)
      settings: SourceProductBaseCode=PS
  HTG : powerlib/Machines/Hydraulic Turbine and Governor  sm="[ 10/3  0.07 ]"  gate="[  0.01  0.97518  -0.1  0.1 ]"  reg="[  0.05  1.163  0.105  0  0.01  ]"  hyd="[  0  2.67  ]"  dref=0  po=0.51299
      settings: SourceProductBaseCode=PS
  Sum2 : Sum  Inputs=+-  InputSameDT=on  SaturateOnIntegerOverflow=on  OutDataTypeStr=Inherit: Same as first input
  Terminator : Terminator
  To Workspace : ToWorkspace  VariableName=delref  SampleTime=-1
  To Workspace1 : ToWorkspace  VariableName=freqref  SampleTime=-1
  Vref : Constant
  wref : Constant
  Pm : Outport  InitialOutput=0
  Vf : Outport  Port=2  InitialOutput=0
  tag scope: d1=global, dw1=global
  wires:
  HTG/2 -> Terminator/1
  Vref/1 -> EXCITATION/1
  m/1 -> Bus Selector/1
  Bus Selector/4 -> HTG/5  "<Rotor speed deviation  dw (pu)>"
  Bus Selector/5 -> To Workspace1/1, [dw1], HTG/4, Sum2/2  "<Output active power   Peo (pu)>"
  Bus Selector/3 -> HTG/3  "<Rotor speed  wm  (pu)>"
  Pref/1 -> HTG/2
  wref/1 -> HTG/1
  HTG/1 -> Pm/1, Sum2/1
  Bus Selector/2 -> EXCITATION/3  "<Stator voltage  vq (pu)>"
  EXCITATION/1 -> Vf/1
  Bus Selector/1 -> EXCITATION/2  "<Stator voltage  vd (pu)>"
  Generic Power System Stabilizer/1 -> EXCITATION/4
  Sum2/1 -> Generic Power System Stabilizer/1
  Bus Selector/6 -> To Workspace/1, [d1]  "<Load angle   delta  (deg)>"

== matlab function IEEE9_16b_2/Relay/MATLAB Function ==
  settings: updateMethod=DISCRETE
  data: Vabc input; Za output; Iabc input; Zb output; Zc output; Zab output; Zbc output; Zca output; Za_3ph output; Zb_3ph output; Zc_3ph output; T1 output; T2 output; T3 output
function [Za, Zb, Zc, Zab, Zbc, Zca, Za_3ph, Zb_3ph, Zc_3ph, T1, T2, T3] = fcn(Vabc, Iabc)
 
persistent init C1 C2 C3 r1 r2 r3 trip1 trip2 trip3 k
if isempty(init)  
    trip1 = false; trip2 = false; trip3 = false;
    Zline = 100*(0.0449 + 1i*2*pi*60*1.01e-3);
    Z0_line = 100*(0.11241 + 1i*60*2.02e-3*2*pi);
    k = (Z0_line - Zline)./Zline;
    Z1 = 0.80*Zline;
    Z2 = 1.2*Zline;
    Z3 = 2*abs(Zline)*exp(1i*80*pi/180);
    C1 = Z1/2; C2 = Z2/2; C3 = Z3/2;
    r1 = abs(C1); r2 = abs(C2); r3 = abs(C3);
    MTA1 = angle(Z1);
    MTA2 = angle(Z2);
    MTA3 = 80*pi/180;
    init = 1;
    
    circle(real(C1),imag(C1),r1)
    circle(real(C2),imag(C2),r2)
    circle(real(C3),imag(C3),r3)
end

Va = Vabc(1); Vb = Vabc(2); Vc = Vabc(3);
Ia = Iabc(1); Ib = Iabc(2); Ic =Iabc(3);
Io = (Ia+Ib+Ic)/3;

Za = Va/(Ia+k*Io);
Zb = Vb/(Ib+k*Io);
Zc = Vc/(Ic+k*Io);
Zab = (Va-Vb)/(Ia-Ib);
Zbc = (Vb-Vc)/(Ib-Ic);
Zca = (Vc-Va)/(Ic-Ia);
Za_3ph = Va/Ia;
Zb_3ph = Vb/Ib;
Zc_3ph = Vc/Ic;

if any([abs(Za-C1),abs(Zb-C1),abs(Zc-C1),abs(Zab-C1),abs(Zbc-C1),abs(Zca-C1),abs(Za_3ph-C1),abs(Zb_3ph-C1),abs(Zc_3ph-C1)] <= r1)
    trip1 = true;
elseif any([abs(Za-C2),abs(Zb-C2),abs(Zc-C2),abs(Zab-C2),abs(Zbc-C2),abs(Zca-C2),abs(Za_3ph-C2),abs(Zb_3ph-C2),abs(Zc_3ph-C2)] <= r2)
    trip2 = true;
elseif any([abs(Za-C3),abs(Zb-C3),abs(Zc-C3),abs(Zab-C3),abs(Zbc-C3),abs(Zca-C3),abs(Za_3ph-C3),abs(Zb_3ph-C3),abs(Zc_3ph-C3)] <= r3)
    trip3 = true;
end

T1 =trip1; T2 = trip2; T3 = trip3;
end
